simulink model "missleFreight"  (Simulink 7.1)
settings: Solver=ode45  StartTime=0.0  StopTime=simTime  FixedStep=t_sim  RelTol=1e-3
values from neighbouring files (symbols this model uses):
  gFin = 2412    [missleTargeting.m]
  gGB = 1/302.7    (= 0.00330360092501)    [missleTargeting.m]
  gGE = .3    (= 0.3)    [missleTargeting.m]
  gSA = 30    [missleTargeting.m]
undefined symbols (not defined in the file or in its folder): C
settings Model: Creator=christopher.rappa  LastModifiedBy=christopher.rappa

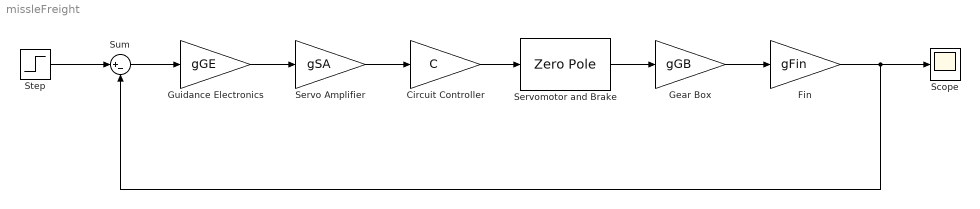
== system missleFreight ==
  Circuit Controller : Gain  Gain=C  ParameterDataType=sfix(16)  ParameterScaling=2^0  OutDataType=sfix(16)  OutScaling=2^0
  Fin : Gain  Gain=gFin  ParameterDataType=sfix(16)  ParameterScaling=2^0  OutDataType=sfix(16)  OutScaling=2^0
  Gear Box : Gain  Gain=gGB  ParameterDataType=sfix(16)  ParameterScaling=2^0  OutDataType=sfix(16)  OutScaling=2^0
  Guidance Electronics : Gain  Gain=gGE  ParameterDataType=sfix(16)  ParameterScaling=2^0  OutDataType=sfix(16)  OutScaling=2^0
  Scope : Scope
  Servo Amplifier : Gain  Gain=gSA  ParameterDataType=sfix(16)  ParameterScaling=2^0  OutDataType=sfix(16)  OutScaling=2^0
  Servomotor and Brake : ZeroPole  Zeros=[]  Poles=[0 1.6 33.8]  Gain=[3.62]
  Step : Step  SampleTime=0
  Sum : Sum  Inputs=|+-  OutDataType=sfix(16)  OutScaling=2^0
  wires:
  Step/1 -> Sum/1
  Sum/1 -> Guidance Electronics/1
  Guidance Electronics/1 -> Servo Amplifier/1
  Gear Box/1 -> Fin/1
  Servomotor and Brake/1 -> Gear Box/1
  Fin/1 -> Sum/2, Scope/1
  Servo Amplifier/1 -> Circuit Controller/1
  Circuit Controller/1 -> Servomotor and Brake/1
